simulink model "flightControlSystem"  (R2024a)
settings: Solver=ode3  StartTime=0  StopTime=TFinal  FixedStep=Ts  RelTol=1e-3  EnableMultiTasking=on
undefined symbols (not defined in the file): codertarget, Controller, DiscIntNeverNeededParam, Discrete, Estimator, g, init, orient_ref, pos_ref, Sensors, Time, Ts, var_acc_angle_N, var_bias_gyr_N, var_gyro_p_N, Vehicle
libraries: simulink x125, slpidlib x35, ctrlSharedLib x12, sharedtransform x10, eeGeneralControl x8, parrotlib x6, shareduavrstlib x1, simulink_need_slupdate x1
(part 10 of 11)

== matlab function flightControlSystem/Control System/Path Planning/MATLAB Function1 ==
  data: u input; forward output; right output; yawgo output; left output; sum_of_region_right output; sum_of_region_forward output; yawcheck output
function [forward,right,yawgo,left,sum_of_region_right,sum_of_region_forward,yawcheck]= fcn(u)



    
        
        % Determine the midpoint of the image along the vertical axis
   
        
        % Set the pixels below the midpoint to black
        %u(midpoint + 10:end, :) = 0;
        
        % Perform noise reduction
        
%         if (filtered_u(1:30,75:85))==1
%             forward=1
%             right=0
%         elseif (filtered_u(58:65,120:150))==1
%             forward=0
%             right=1
%         else
%             forward=0
%             right=0
%         end

%%%%%%%%%%%%%%%%%%%%%%%%%%%%%%%%%%%%%%%%%%%%%%%%%%%%%%%%
        row_range_right = 55:65;
        col_range_right = 130:150;
   
        region_of_interest_right = u(row_range_right, col_range_right);
  
        sum_of_region_right = sum(region_of_interest_right(:))

        %%%%%%%%%%%%%%%%%%%%%%%%%%%%%%%%%%%%%%%%%%%%%%%%%%%%%%
         row_range_forward = 1:20;
         col_range_forward = 75:85;
        
         region_of_interest_forward = u(row_range_forward, col_range_forward);
        
         sum_of_region_forward = sum(region_of_interest_forward(:))


         %%%%%%%%%%%%%%%%%%%%%%%%%%%%%%%%%%%%%%%%%%%%%%%%%%%%%

         row_range_left=55:65;
         col_range_left=1:20;
         region_of_interest_left = u(row_range_left, col_range_left);
        
         sum_of_region_left = sum(region_of_interest_left(:))


%%%%%%%%%%%%%%%%%%%%%%%%%%%%%%%%%%%%%%%%%%%%%%%%%%%%%%
        mid_area=u(59:61,78:82);
        yawcheck=sum(mid_area(:))
        if yawcheck>12
            yawgo=1
        else
            yawgo=0
        end




        %%%%%%%%%%%%%%%%%%%%%%%%%%%%%%%%%%%%%%%%%
%         if u(48:50,80:82)==1 
%             circle_area1=1;
%         else
%             circle_area1=0;
%         end
%       
%         if u(80:82:80:82)==1
%             circle_area2=1
%         else
%             circle_area2=0
%         end
% 
%         if circle_area2 && circle_area1==1
% 
%             land=1;
%         else
%             land=0;
%         end

%%%%%%%%%%%%%%%%%%%%%%%%%%%%%%%%%%%%%%%%%%%%%%%%

        if sum_of_region_right>160
               right=1;
               forward=0;
               left=0;
  
        elseif sum_of_region_forward>190
            forward=1;
            right=0;
            left=0;

        elseif sum_of_region_left>170
            left=1;
            forward=0;
            right=0;
        else
            forward=0;
            right=0;
            left=0;
        end


%         % Define the region of interest for circle detection
%         row_range_circle = [40:80]; 
%         col_range_circle = [60:100]; 
%     
%         % Extract the region of interest for circle detection
%         region_of_interest_circle = u(row_range_circle, col_range_circle);
%     
%         % Calculate the center and radius of the circle
%         center = [length(row_range_circle)/2, length(col_range_circle)/2];
%         radius = min(length(row_range_circle), length(col_range_circle)) / 2;
%     
%         % Generate a circle using the equation of a circle
%         [x, y] = meshgrid(1:length(col_range_circle), 1:length(row_range_circle));
%         circle = (x - center(2)).^2 + (y - center(1)).^2 <= radius^2;
%     
%         % Compare the region of interest with the generated circle
%         similarity = sum(sum(region_of_interest_circle & circle)) / sum(circle(:))
% 
%     
%         % Set a threshold for circle detection (adjust as needed)
%         threshold = 0.7;
%     
%         % If the region of interest is similar to the generated circle, set the land flag
%         if similarity > threshold
%             land = 1
%         else
%             land=0
%         end
end

== matlab function flightControlSystem/Flight Control System/Controller/Position Controller/Position error transformation (Earth to Body frame) ==
  data: yaw input; xy_err_earth input; xy_err_body output
function xy_err_body = fcn(yaw,xy_err_earth)

transformation = [cos(yaw), sin(yaw); -sin(yaw),  cos(yaw)];
xy_err_body = transformation * xy_err_earth;


end

== stateflow chart flightControlSystem/Flight Control System/Path Planning/Chart ==
  settings: initializeOutput=1
  state hover4
    xout = xout-0.0005;
    yout = yout;
    zout = -0.7;
  state right
    xout =xout;
    yout = yout+0.001 ;
    zout = -0.7;
  state go
    xout = xout + 0.003;
    yout = yout ;
    zout = -0.7;
  state hover
    xout = 0.0;
    yout = 0.0;
    zout = -1.0;
  state hover3
    xout = xout;
    yout = yout;
    zout = -0.7;
  state search1
    xout = xout ;
    yout = yout +0.005;
    zout = -0.7;
  state search
    xout = xout;
    yout = yout-0.005 ;
    zout = -0.7;
  state hover6
    xout = xout;
    yout = yout;
    zout = -0.7;
  state hover2
    xout = xout;
    yout = yout;
    zout = -0.7;
  hover4 -> right : [after(1,sec)&&right==1]
  go -> hover4 : [ right==1&&forward==0]
  (default) -> hover
  hover -> go [order 2] : [after(5, sec) && forward==1]
  hover3 -> go : after(3,sec)
  search1 -> hover3 [order 1] : [forward==1]
  hover -> search [order 1] : [after(5, sec) && forward==0]
  search -> hover3 [order 1] : [forward==1]
  hover6 -> search1 : [after(2,sec)&&forward==0]
  search -> hover6 [order 2] : [after(3,sec) &&forward==0]
  search1 -> hover2 [order 2] : [after(3,sec)&&forward==0]
  hover2 -> search : [after(3,sec)&&forward==0]
  data: xout output; yout output; zout output; forward input; right input

== matlab function flightControlSystem/Flight Control System/Path Planning/MATLAB Function ==
  data: u input; xin output; yin output; zin output
function [xin,yin,zin] = fcn(u)

if u(:)==1
    xin=0;
    yin=0;
    zin=-1.0;
else
    xin=0
    yin=0
    zin=-2
end

== matlab function flightControlSystem/Flight Control System/Path Planning/MATLAB Function1 ==
  data: u input; forward output; right output
function [forward,right]= fcn(u)



        [rows, cols] = size(u);
        
     
        
        % Set the pixels below the midpoint to black
        %u(midpoint + 10:end, :) = 0;
        
        % Perform noise reduction
        %filtered_u = medfilt2(u); % Median filtering for noise reduction

%         if (filtered_u(1:30,75:85))==1
%             forward=1
%             right=0
%         elseif (filtered_u(58:65,120:150))==1
%             forward=0
%             right=1
%         else
%             forward=0
%             right=0
%         end
        row_range1 = 50:70;
        col_range1 = 120:150;
   
        region_of_interest1 = u(row_range1, col_range1);
  
        sum_of_region1 = sum(region_of_interest1(:));

        %%%%%%%%%%%%%%%%%%%%%%%%%%%%%%%%%%%%%%%%%%%%%%%%%%%%%%
         row_range = 1:20;
         col_range = 65:75;
        
         region_of_interest = u(row_range, col_range);
        
         sum_of_region = sum(region_of_interest(:));



        

        if sum_of_region1>200
               right=1;
               forward=0;
  

        elseif sum_of_region>200
            forward=1;
            right=0;
        else
            forward=0;
            right=0;

end

== stateflow chart flightControlSystem/Flight Control System/Path Planning/Path Planning1/Chart1 ==
  state hover4
    xout = xout-0.0005;
    yout = yout;
    zout = -0.7;
  state right
    xout =xout;
    yout = yout+0.001 ;
    zout = -0.7;
  state go
    xout = xout + 0.0007;
    yout = yout ;
    zout = -0.7;
  state hover
    xout = 0.0;
    yout = 0.0;
    zout = -1.0;
  state hover3
    xout = xout;
    yout = yout;
    zout = -0.7;
  state search1
    xout = xout ;
    yout = yout +0.0001;
    zout = -0.7;
  state search
    xout = xout;
    yout = yout-0.0001 ;
    zout = -0.7;
  state hover1
    xout = xout;
    yout = yout;
    zout = -0.7;
  state hover2
    xout = xout;
    yout = yout;
    zout = -0.7;
  hover4 -> right : [after(1,sec)&&right==1]
  go -> hover4 : [ right==1&&forward==0]
  (default) -> hover
  59 -> hover
  hover -> go [order 2] : [after(8, sec) && forward==1]
  hover3 -> go : after(3,sec)
  search1 -> hover3 [order 1] : [forward==1]
  hover -> search [order 1] : [after(8, sec) && forward==0]
  search -> hover3 [order 1] : [forward==1]
  hover1 -> search1 : [after(2,sec)&&forward==0]
  search -> hover1 [order 2] : [after(3,sec) &&forward==0]
  search1 -> hover2 [order 2] : [after(3,sec)&&forward==0]
  hover2 -> search : [after(3,sec)&&forward==0]
  data: xout output; yout output; zout output; forward input; right input

== matlab function flightControlSystem/Flight Control System/Path Planning/Path Planning1/MATLAB Function ==
  data: u input; forward output; right output
function [forward,right]= fcn(u)

forward = u(1);
right=u(2);

== matlab function flightControlSystem/Flight Control System/Path Planning/Path Planning1/MATLAB Function1 ==
  data: u input; forward output; right output
function [forward,right]= fcn(u)



        [rows, cols] = size(u);
        
     
        
        % Set the pixels below the midpoint to black
        %u(midpoint + 10:end, :) = 0;
        
        % Perform noise reduction
        filtered_u = medfilt2(u); % Median filtering for noise reduction

%         if (filtered_u(1:30,75:85))==1
%             forward=1
%             right=0
%         elseif (filtered_u(58:65,120:150))==1
%             forward=0
%             right=1
%         else
%             forward=0
%             right=0
%         end
        row_range1 = 50:70;
        col_range1 = 120:150;
   
        region_of_interest1 = filtered_u(row_range1, col_range1);
  
        sum_of_region1 = sum(region_of_interest1(:));

        %%%%%%%%%%%%%%%%%%%%%%%%%%%%%%%%%%%%%%%%%%%%%%%%%%%%%%
         row_range = 1:20;
         col_range = 65:75;
        
         region_of_interest = filtered_u(row_range, col_range);
        
         sum_of_region = sum(region_of_interest(:));



        

        if sum_of_region1>200
               right=1;
               forward=0;
  

        elseif sum_of_region>200
            forward=1;
            right=0;
        else
            forward=0;
            right=0;

end

== matlab function flightControlSystem/Control System/Path Planning/Path Planning/MATLAB Function ==
  data: u input; xin output; yin output; zin output
function [xin,yin,zin] = fcn(u)

if u(:)==1
    xin=0;
    yin=0;
    zin=-1.0;
else
    xin=0
    yin=0
    zin=-2
end

== matlab function flightControlSystem/Control System/Path Planning/Path Planning/MATLAB Function1 ==
  data: u input; forward output; right output
function [forward,right]= fcn(u)



        [rows, cols] = size(u);
        
     
        
        % Set the pixels below the midpoint to black
        %u(midpoint + 10:end, :) = 0;
        
        % Perform noise reduction
        %filtered_u = medfilt2(u); % Median filtering for noise reduction

%         if (filtered_u(1:30,75:85))==1
%             forward=1
%             right=0
%         elseif (filtered_u(58:65,120:150))==1
%             forward=0
%             right=1
%         else
%             forward=0
%             right=0
%         end
        row_range1 = 50:70;
        col_range1 = 120:150;
   
        region_of_interest1 = u(row_range1, col_range1);
  
        sum_of_region1 = sum(region_of_interest1(:));

        %%%%%%%%%%%%%%%%%%%%%%%%%%%%%%%%%%%%%%%%%%%%%%%%%%%%%%
         row_range = 1:20;
         col_range = 65:75;
        
         region_of_interest = u(row_range, col_range);
        
         sum_of_region = sum(region_of_interest(:));



        

        if sum_of_region1>200
               right=1;
               forward=0;
  

        elseif sum_of_region>200
            forward=1;
            right=0;
        else
            forward=0;
            right=0;

end

== stateflow chart flightControlSystem/Control System/Path Planning/Path Planning/Path Planning1/Chart1 ==
  state hover4
    xout = xout-0.0005;
    yout = yout;
    zout = -0.7;
  state right
    xout =xout;
    yout = yout+0.001 ;
    zout = -0.7;
  state go
    xout = xout + 0.0007;
    yout = yout ;
    zout = -0.7;
  state hover
    xout = 0.0;
    yout = 0.0;
    zout = -1.0;
  state hover3
    xout = xout;
    yout = yout;
    zout = -0.7;
  state search1
    xout = xout ;
    yout = yout +0.0001;
    zout = -0.7;
  state search
    xout = xout;
    yout = yout-0.0001 ;
    zout = -0.7;
  state hover1
    xout = xout;
    yout = yout;
    zout = -0.7;
  state hover2
    xout = xout;
    yout = yout;
    zout = -0.7;
  hover4 -> right : [after(1,sec)&&right==1]
  go -> hover4 : [ right==1&&forward==0]
  (default) -> hover
  59 -> hover
  hover -> go [order 2] : [after(8, sec) && forward==1]
  hover3 -> go : after(3,sec)
  search1 -> hover3 [order 1] : [forward==1]
  hover -> search [order 1] : [after(8, sec) && forward==0]
  search -> hover3 [order 1] : [forward==1]
  hover1 -> search1 : [after(2,sec)&&forward==0]
  search -> hover1 [order 2] : [after(3,sec) &&forward==0]
  search1 -> hover2 [order 2] : [after(3,sec)&&forward==0]
  hover2 -> search : [after(3,sec)&&forward==0]
  data: xout output; yout output; zout output; forward input; right input

== matlab function flightControlSystem/Control System/Path Planning/Path Planning/Path Planning1/MATLAB Function ==
  data: u input; forward output; right output
function [forward,right]= fcn(u)

forward = u(1);
right=u(2);

== matlab function flightControlSystem/Control System/Path Planning/Path Planning/Path Planning1/MATLAB Function1 ==
  data: u input; forward output; right output
function [forward,right]= fcn(u)



        [rows, cols] = size(u);
        
     
        
        % Set the pixels below the midpoint to black
        %u(midpoint + 10:end, :) = 0;
        
        % Perform noise reduction
        filtered_u = medfilt2(u); % Median filtering for noise reduction

%         if (filtered_u(1:30,75:85))==1
%             forward=1
%             right=0
%         elseif (filtered_u(58:65,120:150))==1
%             forward=0
%             right=1
%         else
%             forward=0
%             right=0
%         end
        row_range1 = 50:70;
        col_range1 = 120:150;
   
        region_of_interest1 = filtered_u(row_range1, col_range1);
  
        sum_of_region1 = sum(region_of_interest1(:));

        %%%%%%%%%%%%%%%%%%%%%%%%%%%%%%%%%%%%%%%%%%%%%%%%%%%%%%
         row_range = 1:20;
         col_range = 65:75;
        
         region_of_interest = filtered_u(row_range, col_range);
        
         sum_of_region = sum(region_of_interest(:));



        

        if sum_of_region1>200
               right=1;
               forward=0;
  

        elseif sum_of_region>200
            forward=1;
            right=0;
        else
            forward=0;
            right=0;

end

== stateflow chart flightControlSystem/Control System/Path Planning/Chart2 ==
  state hover4
    xout = xout-0.0005;
    yout = yout;
    zout = -0.7;
  state right
    xout =xout;
    yout = yout+0.001 ;
    zout = -0.7;
  state go
    xout = xout + 0.0007;
    yout = yout ;
    zout = -0.7;
  state hover3
    xout = xout;
    yout = yout;
    zout = -0.7;
  state hover
    xout = 0.0;
    yout = 0.0;
    zout = -0.7;
  state search
    xout = xout;
    yout = yout-0.0004 ;
    zout = -0.7;
  state hover1
    xout = xout;
    yout = yout;
    zout = -0.7;
  state hover5
    xout = xout;
    yout = yout;
    zout = -0.7;
  state searchforward
    xout = xout + 0.0004;
    yout = yout ;
    zout = -0.7;
  state search1
    xout = xout ;
    yout = yout +0.0004;
    zout = -0.7;
  state searchforward1
    xout = xout + 0.0004;
    yout = yout ;
    zout = -0.7;
  state hover2
    xout = xout;
    yout = yout;
    zout = -0.7;
  hover4 -> right : [after(2,sec)&&right==1]
  go -> hover4 : [ right==1&&forward==0]
  hover -> hover4 [order 3] : [after(5,sec)&&right==1]
  hover3 -> go : after(3,sec)
  search1 -> hover3 [order 1] : [forward==1]
  hover -> go [order 2] : [after(5, sec) && forward==1]
  (default) -> hover
  searchforward -> hover3 [order 2] : [forward==1]
  search -> hover3 [order 1] : [forward==1]
  hover -> searchforward [order 1] : [after(5, sec) && forward==0 && right==0]
  search -> hover1 [order 2] : [after(3,sec) &&forward==0]
  hover5 -> search : after(3,sec)
  hover1 -> search1 : [after(2,sec)&&forward==0]
  searchforward -> hover5 [order 1] : [after(3,sec)&&forward==0]
  hover2 -> search : [after(3,sec)&&forward==0]
  searchforward -> searchforward1 [order 3] : [yawgo==1]
  search1 -> hover2 [order 2] : [after(6,sec)&&forward==0]
  data: yawgo input; data input; xout output; yout output; zout output; forward input; right input

== stateflow chart flightControlSystem/Control System/Path Planning/Chart3 ==
  state right
    xout =xout;
    yout = yout+0.0005 ;
    zout = -0.7;
  state land2
    xout =xout;
    yout = yout ;
    zout = -0.7;
  state hover4
    xout = xout-0.0001;
    yout = yout;
    zout = -0.7;
    yaw=yaw
  state land1
    xout =xout;
    yout = yout ;
    zout = -0.7;
    finaland=1
  state hover7
    xout = xout;
    yout = yout-0.0002;
    zout = -0.7;
  state land
    xout =xout;
    yout = yout ;
    zout = -0.7;
  state hover8
    xout = xout;
    yout = yout;
    zout = -0.7;
  state yawalign1
    xout = xout ;
    yout = yout ;
    zout = -0.7;
    yaw=yaw+0.0005
  state hover
    xout = 0.0;
    yout = -0.2;
    zout = -0.7;
    yaw=0.5
  state hover6
    xout = xout;
    yout = yout;
    zout = -0.7;
  state yawalign
    xout = xout ;
    yout = yout ;
    zout = -0.7;
    yaw=yaw-0.0005
  state forward
    xout =xout+0.0005;
    yout = yout;
    zout = -0.7;
    yaw=yaw
  right -> hover6 : [yawgo==1&&forward==0]
  land2 -> right : after(2,sec)
  hover4 -> land2 : [right==1&&yawgo==0]
  hover7 -> land1 : [land==1]
  hover8 -> hover4 : after(2,sec)
  land -> hover7 : [after(2,sec)&&land==0]
  (default) -> land [order 2] : [land==1]
  hover -> hover8 [order 2] : [after(5,sec)&&right==1&&yawgo==0]
  (default) -> hover [order 1]
  hover -> ? : [after(5, sec) && forward==0 && right==0&&yawgo==0]
  yawalign -> yawalign1 : [after(10,sec)&&forward==0&&yawgo==1]
  yawalign1 -> yawalign : [after(10,sec)&&forward==0&&yawgo==1]
  hover -> forward [order 1] : [after(5, sec) && forward==1&&yawgo==1]
  hover6 -> yawalign : after(2,sec)
  data: yawgo input; xout output; yout output; zout output; forward input; right input; yaw output; land input; finaland output

== stateflow chart flightControlSystem/Control System/Path Planning/combined ==
  state hover9
    xout = xout-0.0001;
    yout = yout;
    zout = -0.7;
    yaw=yaw
  state right1
    xout =xout;
    yout = yout-0.0005 ;
    zout = -0.7;
  state land4
    xout =xout;
    yout = yout ;
    zout = -0.7;
  state xback5 [commented out]
    xout = xout;
    yout = yout;
    zout = -0.5;
    yaw=yaw+0.0004;
  state hover12
    xout =xout;
    yout = yout ;
    zout = -0.5;
    yaw=yaw;
  state hover11
    xout = xout;
    yout = yout;
    zout = -0.7;
  state xback4
    xout = xout-0.0001;
    yout = yout;
    zout = -0.5;
    yaw=yaw;
  state hover7
    xout = xout;
    yout = yout+0.0002;
    zout = -0.6;
  state land
    xout =xout;
    yout = yout ;
    zout = -0.8;
  state right
    xout =xout;
    yout = yout+0.0005 ;
    zout = -0.5;
    yaw=0;
  state hover8
    xout = xout;
    yout = yout;
    zout = -0.5;
    yaw=yaw;
  state land6
    xout =xout;
    yout = yout ;
    zout = -0.6;
  state go
    xout = xout + 0.0005;
    yout = yout ;
    zout = -0.5;
    yaw=yaw;
  state land1
    xout =xout;
    yout = yout ;
    zout = -0.6;
    finaland=1
  state hover3
    xout = xout;
    yout = yout;
    zout = -0.5;
    yaw=yaw;
  state hover
    xout = 0.0;
    yout = 0;
    zout = -0.7;
    yaw=0;
  state hover5
    xout = xout;
    yout = yout;
    zout = -0.5;
    yaw=yaw;
  state search
    xout = xout;
    yout = yout+0.0001;
    zout = -0.5;
    yaw=yaw;
  state hover1
    xout = xout;
    yout = yout;
    zout = -0.5;
    yaw=yaw;
  state searchforward
    xout = xout + 0.0002;
    yout = yout ;
    zout = -0.5
    yaw=yaw;
  state search1
    xout = xout ;
    yout = yout -0.0002;
    zout = -0.5;
    yaw=yaw;
  state yawalign1
    xout = xout ;
    yout = yout ;
    zout = -0.5;
    yaw=yaw-0.0003
  state hover6
    xout = xout;
    yout = yout;
    zout = -0.5;
    yaw=yaw
  state yawalign
    xout = xout ;
    yout = yout ;
    zout = -0.5;
    yaw=yaw+0.0003
  state hover2
    xout = xout;
    yout = yout;
    zout = -0.5;
    yaw=yaw;
  right -> xback5 [commented out] : [after(1,sec)&&right==0]
  xback5 -> hover12 [commented out] : [after(1.5,sec)&&right==1]
  land4 -> right1 : {after(2,sec)&&yawgo==1}
  hover9 -> land4 : [left==1&yawgo==1]
  hover11 -> hover9 : after(2,sec)
  xback4 -> hover12 : [right==1&&yawgo==1]
  xback4 -> xback5 [commented out] : [after(2,sec)&&right==0&&yawgo==1]
  hover12 -> right : [after(2.5,sec)&&right==1&&yawgo==1]
  go -> hover11 [order 2] : [after(5,sec)&&left==1]
  land -> hover7 : [right==0&&yawgo==1]
  hover8 -> xback4 : after(2,sec)
  hover7 -> land6 : [after(5,sec)&&left==0&&yawgo==1&&right==0]
  right -> land : [after(10,sec)&&right==0&&yawgo==1]
  land6 -> land1 : [after(2,sec)&&yawgo==1&&right==0]
  go -> hover8 [order 1] : [ right==1]
  hover3 -> yawalign [order 2] : [yawgo==1&&forward==0]
  hover3 -> go [order 1] : [after(2,sec)&&forward==1]
  hover -> go [order 2] : [after(5, sec) && forward==1&&yawgo==1]
  (default) -> hover
  yawalign -> hover3 [order 1] : [forward==1&&yawgo==1]
  yawalign1 -> hover3 [order 1] : [forward==1&&yawgo==1]
  search1 -> hover3 [order 1] : [forward==1&&yawgo==1]
  searchforward -> hover3 [order 1] : [forward==1&&yawgo==1]
  search -> hover3 [order 1] : [forward==1&&yawgo==1]
  hover -> hover6 [order 3] : [after(4,sec)&&yawgo==1 &&forward==0]
  hover -> searchforward [order 1] : [after(5, sec) && forward==0 && right==0&&yawgo==0]
  hover5 -> search [order 1] : after(3,sec)
  search -> hover1 [order 2] : [after(12,sec) &&forward==0&&yawgo==0]
  searchforward -> hover5 [order 2] : [after(8,sec)&&forward==0&&yawgo==0]
  hover1 -> search1 [order 1] : [after(2,sec)&&forward==0&&yawgo==0]
  hover5 -> hover6 [order 2] : [yawgo==1&forward==0]
  search -> hover6 [order 3] : [yawgo==1&&forward==0]
  hover2 -> search [order 1] : [after(3,sec)&&forward==0&&yawgo==0]
  hover1 -> hover2 [order 2] : [yawgo==1]
  yawalign -> searchforward [order 2] : [after(5,sec)&&yawgo==0&&forward==0]
  searchforward -> hover6 [order 3] : [yawgo==1&&forward==0]
  yawalign -> yawalign1 [order 3] : [yaw<-0.5&&forward==0&&yawgo==1]
  yawalign1 -> yawalign [order 2] : [yaw>0.5&&forward==0&&yawgo==1]
  search1 -> hover6 [order 3] : [yawgo==1&&forward==0]
  search1 -> hover2 [order 2] : [after(12,sec)&&forward==0&&yawgo==0]
  hover6 -> yawalign : after(2,sec)
  hover2 -> hover6 [order 2] : [after(1,sec)&&yawgo==1]
  data: yawgo input; xout output; yout output; zout output; forward input; right input; yaw output; left input; finaland output

== stateflow chart flightControlSystem/Control System/Path Planning/direct ==
  state hover10 [commented out]
    xout = xout;
    yout = yout-0.0002;
    zout = -0.7;
  state land5 [commented out]
    xout =xout;
    yout = yout ;
    zout = -0.7;
    finaland=1
  state hover9 [commented out]
    xout = xout-0.0001;
    yout = yout;
    zout = -0.7;
    yaw=yaw
  state right1 [commented out]
    xout =xout;
    yout = yout-0.0005 ;
    zout = -0.7;
  state land4 [commented out]
    xout =xout;
    yout = yout ;
    zout = -0.7;
  state land3 [commented out]
    xout =xout;
    yout = yout ;
    zout = -0.7;
  state hover11 [commented out]
    xout = xout;
    yout = yout;
    zout = -0.7;
  state hover4
    xout = xout-0.0001;
    yout = yout;
    zout = -0.7;
    yaw=yaw
  state land2
    xout =xout;
    yout = yout ;
    zout = -0.7;
  state hover7
    xout = xout;
    yout = yout+0.0002;
    zout = -0.7;
  state land
    xout =xout;
    yout = yout ;
    zout = -0.7;
  state right
    xout =xout;
    yout = yout+0.0005 ;
    zout = -0.7;
  state hover8
    xout = xout;
    yout = yout;
    zout = -0.7;
  state land6
    xout =xout;
    yout = yout ;
    zout = -0.7;
  state go
    xout = xout + 0.0005;
    yout = yout ;
    zout = -0.7;
  state land1
    xout =xout;
    yout = yout ;
    zout = -0.5;
    finaland=1
  state hover3
    xout = xout;
    yout = yout;
    zout = -0.7;
  state hover
    xout = 0.0;
    yout =0.0
    zout = -0.7;
    yaw=0.0
  state search
    xout = xout;
    yout = yout+0.0002 ;
    zout = -0.7;
  state hover5
    xout = xout;
    yout = yout;
    zout = -0.7;
  state hover1
    xout = xout;
    yout = yout;
    zout = -0.7;
  state searchforward
    xout = xout + 0.0001;
    yout = yout ;
    zout = -0.7;
  state search1
    xout = xout ;
    yout = yout -0.0004;
    zout = -0.7;
  state hover6
    xout = xout;
    yout = yout;
    zout = -0.7;
  state hover2
    xout = xout;
    yout = yout;
    zout = -0.7;
  land3 -> hover10 [commented out] : [after(2,sec)&&land==0]
  hover10 -> land5 [commented out] : [land==1]
  land3 -> land5 [commented out] : [after(2,sec)&&land==1]
  land4 -> right1 [commented out]
  right1 -> land3 [commented out] : [land==1]
  hover9 -> land4 [commented out] : [left==1]
  hover11 -> hover9 [commented out] : after(2,sec)
  go -> hover11 [commented out] : [after(5,sec)&&left==1]
  hover4 -> land2 : [right==1]
  land2 -> right : [right==1&&yawgo==1]
  land -> hover7 : [after(2,sec)&&right==0&&yawgo==1]
  hover8 -> hover4 : after(2,sec)
  right -> land : [right==0&&yawgo==1]
  hover7 -> land6 : [after(4,sec)&&yawgo==1&&right==0]
  hover -> hover8 [order 1] : [after(5,sec)&&right==1]
  land6 -> land1 : [after(2,sec)&&yawgo==1&&right==0]
  go -> hover8 : [ right==1&&forward==0]
  hover3 -> go : after(3,sec)
  hover -> go [order 3] : [after(5, sec) && forward==1]
  search1 -> hover3 [order 1] : [after(5,sec)&&forward==1]
  (default) -> hover
  searchforward -> hover3 [order 1] : [after(5,sec)&&forward==1]
  search -> hover3 [order 1] : [after(5,sec)&&forward==1]
  hover -> searchforward [order 2] : [after(5, sec) && forward==0 && right==0&&yawgo==0]
  search -> hover1 [order 2] : [after(7,sec) &&forward==0&&yawgo==0]
  hover5 -> search : after(3,sec)
  searchforward -> hover5 [order 2] : [after(5,sec)&&forward==0&&yawgo==0]
  hover1 -> search1 [order 1] : [after(2,sec)&&forward==0&&yawgo==0]
  search -> hover6 [order 3] : [yawgo==1&&forward==0]
  hover2 -> search [order 1] : [after(3,sec)&&forward==0&&yawgo==0]
  hover1 -> hover2 [order 2] : [yawgo==1]
  searchforward -> hover6 [order 3] : [yawgo==1&&forward==0]
  search1 -> hover6 [order 3] : [yawgo==1&&forward==0]
  search1 -> hover2 [order 2] : [after(12,sec)&&forward==0&&yawgo==0]
  hover2 -> hover6 [order 2] : [after(2,sec)&&yawgo==1]
  data: yawgo input; xout output; yout output; zout output; forward input; right input; yaw output; finaland output; left input

== matlab function flightControlSystem/Control System/Path Planning/Subsystem1/MATLAB Function2 ==
  data: u input; forward output; right output; yawgo output; back output; land output; left output; sum_of_region_right output; sum_of_region_forward output; yawcheck output; dy input; dx input
function [forward, right, yawgo,back,land,left, sum_of_region_right, sum_of_region_forward, yawcheck] = fcn(u,dy,dx)


%     scale_forward = 0.005;
%     scale_right =0.004 ;
%     scale_left = 0.005;
%     scale_back=0.004;
  
    scale_forward =1;
    scale_right =1 ;
    scale_left = 1;
    scale_back=1;
  
    

    %%%%%%%%%%%%%%%%%%%%%%%%%%%%%%%%%%%%%%%%%%%%%%%%%%%%%%
    row_range_right = 50:70;
    col_range_right = 90:160;

    region_of_interest_right = u(row_range_right, col_range_right);

    sum_of_region_right = sum(region_of_interest_right(:))

    %%%%%%%%%%%%%%%%%%%%%%%%%%%%%%%%%%%%%%%%%%%%%%%%%%%%%%
    row_range_forward = 1:50;
    col_range_forward = 60:80;

    region_of_interest_forward = u(row_range_forward, col_range_forward);

    sum_of_region_forward = sum(region_of_interest_forward(:))

    %%%%%%%%%%%%%%%%%%%%%%%%%%%%%%%%%%%%%%%%%%%%%%%%%%%%%
    row_range_left = 50:70;
    col_range_left = 1:50;
    region_of_interest_left = u(row_range_left, col_range_left);

    sum_of_region_left = sum(region_of_interest_left(:))

    %%%%%%%%%%%%%%%%%%%%%%%%%%%%%%%%%%%%%%%%%%%%%%%%%%%%%
    row_range_back = 70:120;
    col_range_back = 60:80;
    region_of_interest_back = u(row_range_back, col_range_back);

    sum_of_region_back = sum(region_of_interest_back(:))


    %%%%%%%%%%%%%%%%%%%%%%%%%%%%%%%%%%%%%%%%%%%%%%%%%%%%%%%%%%%
    mid_area = u(59:61, 78:82);
    yawcheck = sum(mid_area(:))
    if yawcheck > 2
        yawgo = 1;
    else
        yawgo = 0;
    end
%      right = scale_right * sum_of_region_right
% 
%     forward = scale_forward * sum_of_region_forward
%      left = scale_left * sum_of_region_left
%      back= scale_back*  sum_of_region_back

    %%%%%%%%%%%%%%%%%%%%%%%%%%%%%%%%%%%%%%%%%%%%%%%%%%%%
    if sum_of_region_right > 160
        right = scale_right * (sum_of_region_right / 160);
        forward = 0;
        left = 0;
        back=0;

    elseif sum_of_region_forward >160
        forward = scale_forward * (sum_of_region_forward / 190);
        right = 0;
        left = 0;
        back=0;

    elseif sum_of_region_left > 160
        left = scale_left * (sum_of_region_left / 160);
        forward = 0;
        right = 0;
        back=0;
    elseif sum_of_region_back > 160
        left = 0;
        forward = 0;
        right = 0;
        back= scale_back* (sum_of_region_left / 200);

  
    else
        forward = 0;
        right = 0;
        left = 0;
        back=0;
    end

    
    if abs(dx)+abs(dy)<0.001;
        

        land=1
    else
        
        land=0.0;
    end
end

== stateflow chart flightControlSystem/Control System/Path Planning/Subsystem1/Chart4 ==
  state go2 [commented out]
    xout=xout+0.0003*forward
    yout=yout+0.004*right
    zout=-0.6
  state Hover
    xout=0
    yout=-0.2
    zout=-0.8
  state go
    xout=xout+0.09*forward-0.09*back
    yout=yout+0.09*right-0.09*left
    zout=-0.6
  state finaland
    finaland=1
  go -> go2 [commented out] : [right>250]
  (default) -> Hover
  Hover -> go : [after(2,sec)]
  go -> finaland : [after(20,sec)&&land==1&&yawgo==1]
  data: back input; left input; right input; forward input; yawgo input; yout output double; xout output double; zout output double; finaland output double; land input

== stateflow chart flightControlSystem/Control System/Path Planning/Subsystem/Chart1 ==
  state go2 [commented out]
    xout=xout+0.0003*forward
    yout=yout+0.004*right
    zout=-0.6
  state go
    xout=0.007*forward
    yout=0.002*right-0.002*left
    zout=-0.8
  state Hover
    xout=xest
    yout=yest
    zout=-0.8
    yaw=0
  state go4 [commented out]
    yaw=yaw+0.0004
  state go3 [commented out]
    y=y+0.09*left
    p=p+0.09*forward
    r=r-0.09*left+0.09*right
  state finaland1 [commented out]
    finaland=1
  state go5
    xout=xout+0.0005*cos(yaw)+0.0005*forward+0.0005*right-0.0005*left
    yout=yout+0.0005*sin(yaw)+0.0005*forward+0.0005*right-0.0005*left
    zout=-0.8
  state finaland [commented out]
    y=0
    p=0
    r=0
  go -> go2 [commented out] : [right>250]
  Hover -> go : [after(2,sec)]
  (default) -> Hover
  go -> go4 [commented out] : [after(5,sec)&&sum_of_region_forward<100]
  go -> go3 [commented out] : [after(7,sec)&&sum_of_region_left>1000]
  go3 -> go [commented out] : [after(5,sec)&&sum_of_region_forward>1000]
  go3 -> finaland [commented out] : [after(10,sec)&&land==1&&yawgo==1&&left<0.1]
  go4 -> go5 [commented out] : [sum_of_region_forward>600]
  (default) -> finaland [commented out] : [after(10,sec)&&land==1&&right<0.01]
  finaland -> finaland1 [commented out] : after(3,sec)
  data: _Y_ input; thetapeak input; sum_of_region_left input; left input; right input; forward input; yawgo input; sum_of_region_right input; sum_of_region_forward input; _X_ input; sum_of_region_back input; back input; finaland output double; land input; yout output double; xout output double; zout output double; yaw output double; yest input; xest input

== matlab function flightControlSystem/Control System/Path Planning/Subsystem/MATLAB Function3 ==
  data: u input; forward output; right output; yawgo output; left output; land output; back output; sum_of_region_right output; sum_of_region_forward output; sum_of_region_left output; sum_of_region_back output; yawcheck output; dy input; dx input
function [forward, right, yawgo,left,land,back, sum_of_region_right, sum_of_region_forward,sum_of_region_left,sum_of_region_back, yawcheck] = fcn(u,dy,dx)

    % Define scaling factors for velocity proportional to region of interest sum
      % Define scaling factors for velocity proportional to region of interest sum
    scale_forward = 1;
    scale_right = 1;
    scale_left = 1;
    scale_back=1;
%     u(50:120,1:160)=0;
%     edgesImg = edge(u, 'Canny');
% 
%     theta = linspace(-90, 89, 180); % Range of angles from -90 to 89 degrees
%     [H, T, R] = hough(u, 'Theta', theta);
%     u(70:120,1:60)=0;
%     % Find peaks in the accumulator matrix
%     peaks = houghpeaks(H, 3);
%     
%     % Display the orientation of the line
%     thetapeak = T(peaks(1,2))    
%     thetapeak=deg2rad(thetapeak)
%     
%     [Gx, Gy] = imgradientxy(u, 'sobel');
%     [gradMag, gradDir] = imgradient(Gx, Gy);
% 
% 
% gradDir(gradDir < 0) = gradDir(gradDir < 0) + 2*pi;
% 
% % Find dominant direction of white regions
% whiteRegionDir = mean(gradDir(u == 1))% Assuming binaryImg is your binary image
% 
% % Convert white region direction to degrees
% whiteRegionDirDegrees = rad2deg(whiteRegionDir)
    %%%%%%%%%%%%%%%%%%%%%%%%%%%%%%%%%%%%%%%%%%%%%%%%%%%%%%
    row_range_right = 50:70;
    col_range_right = 110:160;

    region_of_interest_right = u(row_range_right, col_range_right);

    sum_of_region_right = sum(region_of_interest_right(:))

    %%%%%%%%%%%%%%%%%%%%%%%%%%%%%%%%%%%%%%%%%%%%%%%%%%%%%%
    row_range_forward = 1:50;
    col_range_forward = 60:80;

    region_of_interest_forward = u(row_range_forward, col_range_forward);

    sum_of_region_forward = sum(region_of_interest_forward(:))

    %%%%%%%%%%%%%%%%%%%%%%%%%%%%%%%%%%%%%%%%%%%%%%%%%%%%%
    row_range_left = 50:70;
    col_range_left = 1:50;
    region_of_interest_left = u(row_range_left, col_range_left);

    sum_of_region_left = sum(region_of_interest_left(:))

    %%%%%%%%%%%%%%%%%%%%%%%%%%%%%%%%%%%%%%%%%%%%%%%%%%%%%
    row_range_back = 70:120;
    col_range_back = 60:80;
    region_of_interest_back = u(row_range_left, col_range_back);

    sum_of_region_back = sum(region_of_interest_back(:))


    %%%%%%%%%%%%%%%%%%%%%%%%%%%%%%%%%%%%%%%%%%%%%%%%%%%%%%%%%%%
    mid_area = u(59:61, 78:82);
    yawcheck = sum(mid_area(:))
    if yawcheck > 2
        yawgo = 1;
    else
        yawgo = 0;
    end

    
    forward = scale_forward * (sum_of_region_forward / 170);
    left = scale_left * (sum_of_region_left / 170);


    back= scale_back * (sum_of_region_back / 170);
    right = scale_right * (sum_of_region_right / 170);
    %%%%%%%%%%%%%%%%%%%%%%%%%%%%%%%%%%%%%%%%%%%%%%%%%%%%%
%     if sum_of_region_right > 170
%         right = scale_right * (sum_of_region_right / 170);
%         forward = 0;
%         left = 0;
% 
%     elseif sum_of_region_forward > 190
%         forward = scale_forward * (sum_of_region_forward / 190);
%         right = 0;
%         left = 0;
% 
%     elseif sum_of_region_left > 160
%         left = scale_left * (sum_of_region_left / 160);
%         forward = 0;
%         right = 0;
%     else
%         forward = 0;
%         right = 0;
%         left = 0;
%     end

%     circle_area=u(10:100,80);
%     circle_area1=u(60,30:130);
%     circlesum=sum(sum(circle_area1(:))+sum(circle_area(:)))
%     land=0
%     if circlesum>310
%         land=1
%     else
%         land=0
    
    if abs(dx)+abs(dy)<0.005;
        

        land=1
    else
        
        land=0.0;
end

== stateflow chart flightControlSystem/Control System/Path Planning/Path Planning 2/Chart ==
  state MoveStraight
    during:
    xout=xout+0.000017*x_new;
    yout=yout+0.000017*y_new;
    zout=zout;
  state MoveStraight1 [commented out]
    during:
    yaw=yaw+0.0003
  state MoveStraight2 [commented out]
    during:
    xout=xout
    yout=yout
    zout=-0.7
  state Hover
    entry:
    xout=0;
    yout=-0.2;
    zout=-0.7;
    yaw=0;
  state MoveStraight3 [commented out]
    during:
    xout=xout+0.00002*x_new;
    yout=yout+0.00002*y_new;
    zout=zout;
  state land
    finaland=1
  state land1
    xout=xout+0.00002*x_new;
    yout=yout+0.00002*y_new;
    zout=zout;
  (default) -> Hover
  MoveStraight -> MoveStraight1 [commented out] : [abs(ang)<20]
  Hover -> MoveStraight : [after(3,sec)]
  MoveStraight1 -> MoveStraight2 [commented out] : [after(4,sec)&&abs(ang)>65]
  MoveStraight -> land1 : [after(8,sec)&&abs(dx+dy)<0.0001]
  MoveStraight2 -> MoveStraight3 [commented out] : [after(3,sec)&&abs(ang)>60]
  land1 -> land : [after(5,sec)&abs(dx+dy)<0.0001]
  data: finaland output; ang input; sum_pixels input; xestim input; yestim input; y_new input; xout output single; yout output single; zout output single; x_new input; yaw output; dy input; dx input

== matlab function flightControlSystem/Control System/Path Planning/Path Planning 2/MATLAB Function ==
  data: in input; ang output; b output; x_new output; y_new output; sum_pixels output
function [ang, b, x_new, y_new,sum_pixels] = calculate_ang(in)
    ang = 0;
     b = imbinarize(in);
% b=in;
    for row =100:120
        for col = 1:100
            b(row, col) = 0;
        end
    end
    for row =1:120
        for col = 1:55
            b(row, col) = 0;
        end
    end

    input = b;
    N = 1;
    out = zeros(2, N);
    m00 = zeros(1, N);
    m01 = zeros(1, N);
    m10 = zeros(1, N);
    
    [r, c] = size(input);
    
    for row = 1:r
        for col = 1:c
            if input(row, col) ~= 0 % on object pixel
               m10(input(row, col)) = row * 1 + m10(input(row, col)); 
               m01(input(row, col)) = col * 1 + m01(input(row, col));
               m00(input(row, col)) = m00(input(row, col)) + 1;
            end
        end
    end

    for i = 1:N
        if m00(i) ~= 0  % Check if m00 is not zero to avoid division by zero
            out(2, i) = m10(i) / m00(i);
            out(1, i) = m01(i) / m00(i);
        else
            out(2, i) = 0; % Assign default value when m00 is zero
            out(1, i) = 0; % Assign default value when m00 is zero
        end
    end
    
    x_new = out(1, 1);
    y_new = out(2, 1);
    
    if x_new ~= 0  % Check if x_new is not zero to avoid division by zero
        x_new = x_new - 80
        y_new = 60 - y_new
        ang = rad2deg(atan(y_new / x_new))
    else
        ang = 0; % Assign default angle when x_new is zero
    end

    sum_pixels=sum(b(:))
end

== stateflow chart flightControlSystem/Control System/Path Planning/Subsystem2/Chart1 ==
  state MoveStraight
    during:
    xout=xout+0.009*x_new;
    yout=yout+0.009*y_new;
    zout=zout;
  state Hover
    entry:
    xout=0.0;
    yout=0.0;
    zout=-0.7;
  state MoveStraight4
    during:
    xout=xout+0.009*x_new;
    yout=yout+0.009*y_new;
    zout=zout+0.000001*(sum_pixels);
  state land
    finaland=1
  (default) -> Hover
  Hover -> MoveStraight : [after(2,sec)]
  MoveStraight4 -> MoveStraight [order 1] : [sum_pixels<800 ]
  MoveStraight -> MoveStraight4 : [sum_pixels>800&&centroid_dist<45]
  MoveStraight4 -> land [order 2] : [zout>-0.1]
  data: ang input; sum_pixels input; centroid_dist input; xestim input; yestim input; y_new input; xout output single; yout output single; zout output single; x_new input; dy input; dx input; s local; finaland output

== matlab function flightControlSystem/Image Processing System/MATLAB Function ==
  data: x_new output; y_new output; xd_new output; yd_new output; xdd_new output; ydd_new output; sum_pixels output; centroid_dist output; ang output; b output; b input
function [x_new, y_new, xd_new, yd_new, xdd_new, ydd_new, sum_pixels, centroid_dist, ang, b] = trackMovement(b)
    persistent x_old y_old xd_old yd_old; % Persistent variables to store previous states
    
    if isempty(x_old)
        x_old = 0;
        y_old = 0;
        xd_old = 0;
        yd_old = 0;
    end
    dt=0.001
    % Calculate current state (position, angle, etc.) using calculate_ang function
    [ang, b, x_new, y_new, sum_pixels, centroid_dist] = calculate_ang(b);
    
    % Calculate velocity (current derivative of position)
    yd_new = (x_new - x_old)/dt
    xd_new = (y_new - y_old)/dt
    
    % Calculate acceleration (current derivative of velocity)
    xdd_new = (xd_new - xd_old)/dt
    ydd_new = (yd_new - yd_old)/dt
    
    % Update old positions and velocities for the next call
    x_old = x_new;
    y_old = y_new;
    xd_old = xd_new;
    yd_old = yd_new;
end


function [ang, b, x_new, y_new,sum_pixels,centroid_dist] = calculate_ang(in)
    ang = 0;
    % b = imbinarize(in);
    b=in;
    
    input = b;
    N = 1;
    out = zeros(2, N);
    m00 = zeros(1, N);
    m01 = zeros(1, N);
    m10 = zeros(1, N);
    
    [r, c] = size(input);
    
    for row = 1:r
        for col = 1:c
            if input(row, col) ~= 0 % on object pixel
               m10(input(row, col)) = row * 1 + m10(input(row, col)); 
               m01(input(row, col)) = col * 1 + m01(input(row, col));
               m00(input(row, col)) = m00(input(row, col)) + 1;
            end
        end
    end

    for i = 1:N
        if m00(i) ~= 0  % Check if m00 is not zero to avoid division by zero
            out(2, i) = m10(i) / m00(i);
            out(1, i) = m01(i) / m00(i);
        else
            out(2, i) = 0; % Assign default value when m00 is zero
            out(1, i) = 0; % Assign default value when m00 is zero
        end
    end
    
    x_new = out(1, 1)
    y_new = out(2, 1)
    
    if x_new ~= 0  % Check if x_new is not zero to avoid division by zero
        x_new = x_new - 80
        y_new = 60 - y_new
        ang = rad2deg(atan(y_new / x_new))
    else
        ang = 0; % Assign default angle when x_new is zero
    end
    mid_area1=b(45:75,50:100);
    centroid_dist = sqrt((x_new)^2 + (y_new)^2)

    
    sum_pixels=sum(mid_area1(:))
end

== matlab function flightControlSystem/Image Processing System1/MATLAB Function ==
  data: in input; ang output; b output; x_new output; y_new output; sum_pixels output
function [ang, b, x_new, y_new,sum_pixels] = calculate_ang(in)
    ang = 0;
     b = imbinarize(in);
% b=in;
    for row =100:120
        for col = 1:100
            b(row, col) = 0;
        end
    end
    for row =1:120
        for col = 1:55
            b(row, col) = 0;
        end
    end

    input = b;
    N = 1;
    out = zeros(2, N);
    m00 = zeros(1, N);
    m01 = zeros(1, N);
    m10 = zeros(1, N);
    
    [r, c] = size(input);
    
    for row = 1:r
        for col = 1:c
            if input(row, col) ~= 0 % on object pixel
               m10(input(row, col)) = row * 1 + m10(input(row, col)); 
               m01(input(row, col)) = col * 1 + m01(input(row, col));
               m00(input(row, col)) = m00(input(row, col)) + 1;
            end
        end
    end

    for i = 1:N
        if m00(i) ~= 0  % Check if m00 is not zero to avoid division by zero
            out(2, i) = m10(i) / m00(i);
            out(1, i) = m01(i) / m00(i);
        else
            out(2, i) = 0; % Assign default value when m00 is zero
            out(1, i) = 0; % Assign default value when m00 is zero
        end
    end
    
    x_new = out(1, 1);
    y_new = out(2, 1);
    
    if x_new ~= 0  % Check if x_new is not zero to avoid division by zero
        x_new = x_new - 80
        y_new = 60 - y_new
        ang = rad2deg(atan(y_new / x_new))
    else
        ang = 0; % Assign default angle when x_new is zero
    end

    sum_pixels=sum(b(:))
end

== matlab function flightControlSystem/Image Processing System1/MATLAB Function1 ==
  data: R input; BW output; G input; B input
function BW  = createMask(R,G,B)
    % Convert RGB image to chosen color space
    I = cat(3, R, G, B);

    % Define thresholds for each channel
    channel1Min = 108.000;
    channel1Max = 216.000;
    channel2Min = 141.000;
    channel2Max = 250.000;
    channel3Min = 203.000;
    channel3Max = 255.000;

    % Create mask based on chosen histogram thresholds
    BW = (I(:,:,1) >= channel1Min) & (I(:,:,1) <= channel1Max) & ...
         (I(:,:,2) >= channel2Min) & (I(:,:,2) <= channel2Max) & ...
         (I(:,:,3) >= channel3Min) & (I(:,:,3) <= channel3Max);
end

== matlab function flightControlSystem/Control System/Path Planning/Subsystem2/MATLAB Function2 ==
  data: u input; forward output; right output
function [forward,right]= fcn(u)

forward = u(1);
right=u(2);

== stateflow chart flightControlSystem/Control System/Path Planning/Subsystem3/Chart ==
  state MoveStraight
    during:
    xout=xout+0.009*x_new;
    yout=yout+0.009*y_new;
    zout=zout;
  state Hover
    entry:
    xout=0.0;
    yout=0.0;
    zout=-0.7;
  state MoveStraight4
    during:
    xout=xout+0.009*x_new;
    yout=yout+0.009*y_new;
    zout=zout+0.000001*(sum_pixels);
  state land
    finaland=1
  (default) -> Hover
  Hover -> MoveStraight : [after(2,sec)]
  MoveStraight4 -> MoveStraight [order 1] : [sum_pixels<800 ]
  MoveStraight -> MoveStraight4 : [sum_pixels>800&&centroid_dist<45]
  MoveStraight4 -> land [order 2] : [zout>-0.1]
  data: ang input; sum_pixels input; centroid_dist input; xestim input; yestim input; y_new input; xout output single; yout output single; zout output single; x_new input; dy input; dx input; s local; finaland output

== matlab function flightControlSystem/Image Processing System/MATLAB Function1 ==
  data: R input; BW output; G input; B input
function BW  = createMask(R,G,B)
    % Convert RGB image to chosen color space
    I = cat(3, R, G, B);

    % Define thresholds for each channel
    channel1Min = 108.000;
    channel1Max = 216.000;
    channel2Min = 141.000;
    channel2Max = 250.000;
    channel3Min = 203.000;
    channel3Max = 255.000;

    % Create mask based on chosen histogram thresholds
    BW = (I(:,:,1) >= channel1Min) & (I(:,:,1) <= channel1Max) & ...
         (I(:,:,2) >= channel2Min) & (I(:,:,2) <= channel2Max) & ...
         (I(:,:,3) >= channel3Min) & (I(:,:,3) <= channel3Max);
end

== matlab function flightControlSystem/Image Processing System/MATLAB Function2 ==
  data: R input; BW output; G input; B input
function BW  = createMask(R,G,B)
    % Convert RGB image to chosen color space
    I = cat(3, R, G, B);

    % Define thresholds for each channel
    channel1Min = 108.000;
    channel1Max = 216.000;
    channel2Min = 141.000;
    channel2Max = 250.000;
    channel3Min = 203.000;
    channel3Max = 255.000;

    % Create mask based on chosen histogram thresholds
    BW = (I(:,:,1) >= channel1Min) & (I(:,:,1) <= channel1Max) & ...
         (I(:,:,2) >= channel2Min) & (I(:,:,2) <= channel2Max) & ...
         (I(:,:,3) >= channel3Min) & (I(:,:,3) <= channel3Max);
end

== stateflow chart flightControlSystem/Control System/Path Planning/line follow ==
  state MoveStraight
    during:
    xout=xout+0.00002*x_new;
    yout=yout+0.00002*y_new;
    zout=zout;
  state MoveStraight1 [commented out]
    during:
    yaw=yaw+0.0003
  state MoveStraight2 [commented out]
    during:
    xout=xout
    yout=yout
    zout=-0.7
  state Hover
    entry:
    xout=0;
    yout=0;
    zout=-0.7;
  state MoveStraight3 [commented out]
    during:
    xout=xout+0.00002*x_new;
    yout=yout+0.00002*y_new;
    zout=zout;
  state land1
    xout=xout+0.00002*x_new;
    yout=yout+0.00002*y_new;
    zout=zout;
    s=(abs(dx)+abs(dy))
  state land
    zout=-0.9
  state land2
    finaland=1
  (default) -> Hover
  MoveStraight -> MoveStraight1 [commented out] : [abs(ang)<20]
  Hover -> MoveStraight : [after(3,sec)]
  MoveStraight1 -> MoveStraight2 [commented out] : [after(4,sec)&&abs(ang)>65]
  MoveStraight -> land1 : [after(8,sec)&&abs(dx+dy)<0.0001]
  MoveStraight2 -> MoveStraight3 [commented out] : [after(3,sec)&&abs(ang)>60]
  land1 -> land : [after(8,sec)&&s<0.003]
  land -> land2 : after(3,sec)
  data: finaland output; ang input; sum_pixels input; xestim input; yestim input; y_new input; xout output single; yout output single; zout output single; x_new input; dy input; dx input; s local
